simulink model "Mdl_Dim"  (R2024b)
settings: Solver=FixedStepDiscrete  StartTime=0.0  StopTime=10.0  FixedStep=0.1  RelTol=1e-3  EnableMultiTasking=on
values from neighbouring files (symbols this model uses):
  DEFAULT_MODE = mpt.Parameter    [Mdl_Dim_DD.m]
  DEFAULT_STEP = mpt.Parameter    [Mdl_Dim_DD.m]
  Mdl_Dim_cTaskPeriod = mpt.Parameter    [Mdl_Dim_rte_types.m]
  RTE_E_MAX_AGE_EXCEEDED = mpt.Parameter    [Mdl_Dim_rte_types.m]
  RTE_E_NEVER_RECEIVED = mpt.Parameter    [Mdl_Dim_rte_types.m]
  STATUS_OFF = mpt.Parameter    [Mdl_Dim_DD.m]
  STATUS_ON = mpt.Parameter    [Mdl_Dim_DD.m]
  SWITCHING_MECHANISM = mpt.Parameter    [Mdl_Dim_DD.m]
  ZERO_VAL = mpt.Parameter    [Mdl_Dim_DD.m]
undefined symbols (not defined in the file or in its folder): AppModule, CAN_COMUN_ACTIVE, CAN_COMUN_FAIL, CAN_VAL_OFF, CAN_VAL_ON, ChannelID, CLUSTER_ACTIVE, DAYNIGHT_STS_NOTRequire, DIAG_NCTRL, DIM_DAY_MODE, DIM_NIGHT_MODE, DOWN_THRESH_1SW, DrvRec_Rheo_down_Long_Press, DrvRec_Rheo_down_Short_Press, DrvRec_Rheo_up_Long_Press, DrvRec_Rheo_Up_Short_Press, DW_EVENT, DW_ON, eAppMdl_type_instance, eDayNightModeIn, eIllumination_levelIn, eSIGNAL_MISSING, eSIGNAL_NEVER_RECEIVED, eSleepSt_type_instance, FALSE, GetPwmDirect, GetPwmWithTime, GetPwmWithTimeExp, IgnOn, INDEX_MCUID0340, INDEX_MCUID0341, INDEX_MCUID0430, IoHwAb_PwmSignalIdType_type_instance, l_Wheel_Down_ParamArray, l_Wheel_Up_ParamArray, MAX_UINT16, MAXHOLD, MINHOLD, NETWORK_NORMAL, NETWORK_SLEEP, NETWORK_STANDALONE, NONE, NVM_Adapter_SetNVM_RheostatDayStep, NVM_Adapter_SetNVM_RheostatDayStepU1, NVM_Adapter_SetNVM_RheostatDayStepU2, NVM_Adapter_SetNVM_RheostatDayStepU3, NVM_Adapter_SetNVM_RheostatNightStep, NVM_Adapter_SetNVM_RheostatNightStepU1, NVM_Adapter_SetNVM_RheostatNightStepU2, NVM_Adapter_SetNVM_RheostatNightStepU3, OpeModeRheostatChange, pJustRcvdStatus, pNvmData, POS_MAX, POS_MIN, RHEO_1SW_TYPE, RHEO_2SW_TYPE, RHEO_SOFTSW_TYPE, RHEO_VALUE_FIVE_U16, RHEO_VALUE_ONE_BOOL ... (+48)
libraries: simulink x65
(part 4 of 4)

== matlab function Mdl_Dim/Mdl_Dim_Task_sys/Subsystem/Input_Process/Switch Type//2 Switch Type//Soft Switch Type/RHEO_1SW_TYPE_AND_RHEO_2SW_TYPE/Rheostat Switch Status Determination ==
  data: RHUP_Dbc_Status input; RheostatCond input; RHDW_Dbc_Status input; RheostatSwstatus output uint8; STATE_ON parameter; UP_ON parameter; Prevrheoswstatus input; VAL_ON parameter; VAL_OFF parameter; DW_ON parameter; IgnOn parameter; STATE_OFF parameter; UNKNOWN parameter; UNKNOWNSTATUS parameter; TRUE parameter; FALSE parameter
function RheostatSwstatus = fcn(RHUP_Dbc_Status, RheostatCond, RHDW_Dbc_Status, STATE_ON, UP_ON, Prevrheoswstatus, VAL_ON, VAL_OFF, DW_ON, IgnOn, STATE_OFF, UNKNOWN, UNKNOWNSTATUS, TRUE, FALSE)

aVarTruthTableCondition_1 = false;
aVarTruthTableCondition_2 = false;
aVarTruthTableCondition_3 = false;


% condition 2

aVarTruthTableCondition_1 = logical(( (RheostatCond == TRUE) && (RHUP_Dbc_Status == STATE_OFF) && (RHDW_Dbc_Status == STATE_OFF) ));

% condition 6

aVarTruthTableCondition_2 = logical(( (RheostatCond == TRUE) && (RHUP_Dbc_Status == STATE_ON) && ((Prevrheoswstatus == VAL_OFF) || (Prevrheoswstatus == UP_ON) || (Prevrheoswstatus == DW_ON)) ));

% condition 7

aVarTruthTableCondition_3 = logical(( (RheostatCond == TRUE) && (RHUP_Dbc_Status == STATE_OFF) && (RHDW_Dbc_Status == STATE_ON) && ((Prevrheoswstatus == VAL_OFF) || (Prevrheoswstatus == UP_ON) || (Prevrheoswstatus == DW_ON)) ));

if (aVarTruthTableCondition_1)
    aFcnTruthTableAction_2();
elseif (aVarTruthTableCondition_2)
    aFcnTruthTableAction_3();
elseif (aVarTruthTableCondition_3)
    aFcnTruthTableAction_4();
else % Default
    aFcnTruthTableAction_1();
end

function aFcnTruthTableAction_1()

% RhesostatSwitch status

RheostatSwstatus = UNKNOWNSTATUS;

function aFcnTruthTableAction_2()

% RhesostatSwitch status

RheostatSwstatus = VAL_OFF;

function aFcnTruthTableAction_3()

% RhesostatSwitch status

RheostatSwstatus = UP_ON;

function aFcnTruthTableAction_4()

% RhesostatSwitch status

RheostatSwstatus = DW_ON;

== matlab function Mdl_Dim/Mdl_Dim_Task_sys/Subsystem/Input_Process/Switch Type//2 Switch Type//Soft Switch Type/Night_Rheostat_Step_Determination ==
  data: Day_Night_status input; RheostatUpEvent input; RheostatDwEvent input; DIM_DAY_MODE parameter; DIM_NIGHT_MODE parameter; RTE_E_MAX_AGE_EXCEEDED parameter; MINHOLD parameter; MAXHOLD parameter; NVM_RheostatNightStep output; Prev_NVM_RheostatDayStep input; UP_EVENT parameter; NONE parameter; DW_EVENT parameter; NightChangeStatus output; TailStatus input; Get_RheostatNightStep_Val input; TRUE parameter; FALSE parameter; MCUID0341 data_store_memory
function [NVM_RheostatNightStep, NightChangeStatus] = fcn(Day_Night_status, RheostatUpEvent, RheostatDwEvent, DIM_DAY_MODE, DIM_NIGHT_MODE, RTE_E_MAX_AGE_EXCEEDED, MINHOLD, MAXHOLD, Prev_NVM_RheostatDayStep, UP_EVENT, NONE, DW_EVENT, TailStatus, Get_RheostatNightStep_Val, TRUE, FALSE)

aVarTruthTableCondition_1 = false;
aVarTruthTableCondition_2 = false;
aVarTruthTableCondition_3 = false;
aVarTruthTableCondition_4 = false;
aVarTruthTableCondition_5 = false;
aVarTruthTableCondition_6 = false;
aVarTruthTableCondition_7 = false;
aVarTruthTableCondition_8 = false;


% Night status, Up_Event and
% NVM night step >= MAXHOLD(21)

aVarTruthTableCondition_1 = logical(((Day_Night_status  == DIM_NIGHT_MODE) && (RheostatUpEvent == UP_EVENT) && (Get_RheostatNightStep_Val >= MAXHOLD)));

% Night status,Up_Event and NVM night step < MAXHOLD(21)

aVarTruthTableCondition_2 = logical(((Day_Night_status  == DIM_NIGHT_MODE) && (RheostatUpEvent == UP_EVENT) && (Get_RheostatNightStep_Val < MAXHOLD)));

% Night status,DW_Event and NVM night step = 0

aVarTruthTableCondition_3 = logical(((Day_Night_status  == DIM_NIGHT_MODE) && (RheostatUpEvent == NONE) && (RheostatDwEvent == DW_EVENT)&& (Get_RheostatNightStep_Val == MINHOLD)));

% Night status,DW_Event and NVM night step > 0

aVarTruthTableCondition_4 = logical(((Day_Night_status  == DIM_NIGHT_MODE) && (RheostatUpEvent == NONE) && (RheostatDwEvent == DW_EVENT)&& (Get_RheostatNightStep_Val > MINHOLD)));

% Day status, Up_Event and
% NVM night step >= MAXHOLD(21)

aVarTruthTableCondition_5 = logical(((Day_Night_status  == DIM_DAY_MODE) &&(MCUID0341  == TRUE) &&  (TailStatus  == TRUE) && (RheostatUpEvent == UP_EVENT) && (Get_RheostatNightStep_Val >= MAXHOLD)));

% Day status,Up_Event and NVM night step < MAXHOLD(21)

aVarTruthTableCondition_6 = logical(((Day_Night_status  == DIM_DAY_MODE)&&(MCUID0341  == TRUE) &&  (TailStatus  == TRUE) && (RheostatUpEvent == UP_EVENT) && (Get_RheostatNightStep_Val < MAXHOLD)));

% Day status,DW_Event and NVM night step = 0

aVarTruthTableCondition_7 = logical(((Day_Night_status  == DIM_DAY_MODE)  &&(MCUID0341  == TRUE) &&  (TailStatus  == TRUE) && (RheostatUpEvent == NONE) && (RheostatDwEvent == DW_EVENT)&& (Get_RheostatNightStep_Val == MINHOLD)));

% Day status,DW_Event and NVM night step > 0

aVarTruthTableCondition_8 = logical(((Day_Night_status  == DIM_DAY_MODE) &&(MCUID0341  == TRUE) &&  (TailStatus  == TRUE) && (RheostatUpEvent == NONE) && (RheostatDwEvent == DW_EVENT)&& (Get_RheostatNightStep_Val > MINHOLD)));

if (aVarTruthTableCondition_1)
    aFcnTruthTableAction_1();
elseif (aVarTruthTableCondition_2)
    aFcnTruthTableAction_2();
elseif (aVarTruthTableCondition_3)
    aFcnTruthTableAction_3();
elseif (aVarTruthTableCondition_4)
    aFcnTruthTableAction_4();
elseif (aVarTruthTableCondition_5)
    aFcnTruthTableAction_1();
elseif (aVarTruthTableCondition_6)
    aFcnTruthTableAction_2();
elseif (aVarTruthTableCondition_7)
    aFcnTruthTableAction_3();
elseif (aVarTruthTableCondition_8)
    aFcnTruthTableAction_4();
else % Default
    aFcnTruthTableAction_5();
end

function aFcnTruthTableAction_1()

    % NVM_RheostatDayStep

    NVM_RheostatNightStep = MAXHOLD;
    NightChangeStatus = FALSE;

function aFcnTruthTableAction_2()

    % NVM_RheostatDayStep

    NVM_RheostatNightStep = Prev_NVM_RheostatDayStep +1;
    NightChangeStatus = TRUE;

function aFcnTruthTableAction_3()

    % NVM_RheostatDayStep

    NVM_RheostatNightStep = MINHOLD
    NightChangeStatus = FALSE;

function aFcnTruthTableAction_4()

    % NVM_RheostatDayStep

    NVM_RheostatNightStep = Prev_NVM_RheostatDayStep-1;
    NightChangeStatus = TRUE;

function aFcnTruthTableAction_5()


    NVM_RheostatNightStep = Prev_NVM_RheostatDayStep;
    NightChangeStatus = FALSE;

== matlab function Mdl_Dim/Mdl_Dim_Task_sys/Subsystem/Input_Process/Switch Type//2 Switch Type//Soft Switch Type/RHEO_1SW_TYPE_AND_RHEO_2SW_TYPE/Subsystem/Truth Table ==
  data: RHUP_RawIn_Val output; RHEO_SW_IN_ADIN_Val input; RHDW_RawIn_Val output; VAL_ONE parameter; UP_THRESH_1SW parameter; DOWN_THRESH_1SW parameter; TRUE parameter; FALSE parameter
function [RHUP_RawIn_Val, RHDW_RawIn_Val] = fcn(RHEO_SW_IN_ADIN_Val, VAL_ONE, UP_THRESH_1SW, DOWN_THRESH_1SW, TRUE, FALSE)

aVarTruthTableCondition_1 = false;
aVarTruthTableCondition_2 = false;


% UP ON condition

aVarTruthTableCondition_1 = logical((RHEO_SW_IN_ADIN_Val < UP_THRESH_1SW));

% Down ON condition

aVarTruthTableCondition_2 = logical(( (RHEO_SW_IN_ADIN_Val >= UP_THRESH_1SW) && (RHEO_SW_IN_ADIN_Val < DOWN_THRESH_1SW)));

if (aVarTruthTableCondition_1)
    aFcnTruthTableAction_1();
elseif (aVarTruthTableCondition_2)
    aFcnTruthTableAction_2();
else % Default
    aFcnTruthTableAction_3();
end

function aFcnTruthTableAction_1()

% UP ON state

RHUP_RawIn_Val = TRUE;
RHDW_RawIn_Val = FALSE;

function aFcnTruthTableAction_2()

% DW ON state

RHDW_RawIn_Val = TRUE;
RHUP_RawIn_Val = FALSE;

function aFcnTruthTableAction_3()

% UP and DW OFF state

RHDW_RawIn_Val = FALSE;
RHUP_RawIn_Val = FALSE;

== matlab function Mdl_Dim/Mdl_Dim_Task_sys/Subsystem/Input_Process/Thumb Wheel Type/Rheostat_Step_Determination ==
  data: RheostatCond_state input; l_Wheel_RheostatStep data_store_memory; l_Wheel_RheostatChange data_store_memory; RHEO_WHEEL_STEP_INVALID parameter; RHEO_WHEEL_POS_UNDECIDED parameter; WheelPosition input; VAL_ZERO parameter; VAL_ONE parameter; l_WheelVolRatioMon_u8 data_store_memory; VAL_UNDECIDED parameter; l_AveWheelVolRaitoVal_u8 input
function fcn(RheostatCond_state, RHEO_WHEEL_STEP_INVALID, RHEO_WHEEL_POS_UNDECIDED, WheelPosition, VAL_ZERO, VAL_ONE, VAL_UNDECIDED, l_AveWheelVolRaitoVal_u8)

aVarTruthTableCondition_1 = false;
aVarTruthTableCondition_2 = false;
aVarTruthTableCondition_3 = false;


% RheostatStep is INVALID and Wheel Position Undecided

aVarTruthTableCondition_1 = logical((l_Wheel_RheostatStep == RHEO_WHEEL_STEP_INVALID) && (WheelPosition ==RHEO_WHEEL_POS_UNDECIDED));

% RheostatStep is INVALID and Wheel Position not equal to Undecided

aVarTruthTableCondition_2 = logical((l_Wheel_RheostatStep == RHEO_WHEEL_STEP_INVALID) && (WheelPosition ~=RHEO_WHEEL_POS_UNDECIDED));

% RheostatStep not equal to INVALID and Wheel Position not equal to Undecided

aVarTruthTableCondition_3 = logical((RheostatCond_state == VAL_ONE) && (l_Wheel_RheostatStep ~= RHEO_WHEEL_STEP_INVALID) && (WheelPosition ~= l_Wheel_RheostatStep));

if (aVarTruthTableCondition_1)
    aFcnTruthTableAction_1();
elseif (aVarTruthTableCondition_2)
    aFcnTruthTableAction_2();
elseif (aVarTruthTableCondition_3)
    aFcnTruthTableAction_3();
else % Default
    aFcnTruthTableAction_4();
end

function aFcnTruthTableAction_1()

% RheostatStep is INVALID and RheostatChange False

l_Wheel_RheostatStep = RHEO_WHEEL_STEP_INVALID;
l_Wheel_RheostatChange = VAL_ZERO;

function aFcnTruthTableAction_2()

% RheostatStep is Valid and RheostatChange False

l_Wheel_RheostatStep = WheelPosition;
l_Wheel_RheostatChange = VAL_ZERO;
l_WheelVolRatioMon_u8 = VAL_UNDECIDED;

function aFcnTruthTableAction_3()

% RheostatStep is Valid and RheostatChange true

l_Wheel_RheostatStep = WheelPosition;
l_Wheel_RheostatChange = VAL_ONE;
l_WheelVolRatioMon_u8 = l_AveWheelVolRaitoVal_u8;

function aFcnTruthTableAction_4()

% No Change

l_Wheel_RheostatStep = l_Wheel_RheostatStep;
l_Wheel_RheostatChange = VAL_ZERO;
l_WheelVolRatioMon_u8 = l_AveWheelVolRaitoVal_u8;

== matlab function Mdl_Dim/Mdl_Dim_Task_sys/Subsystem/Input_Process/Subsystem/Rheostat_Control_Enable_Condition_Determination ==
  data: TFTDisplayOn input; Ignstatus input; TailStatus_Val input; DIM_NIGHT_MODE parameter; RheostatCond_state output; TFT_DISPLAY_ON parameter; UNKNOWNSTATUS parameter; VAL_OFF parameter; DAYNIGHT_STS_NOTRequire parameter; IlumDayNightStatus input; DIM_DAY_MODE parameter; VAL_ON parameter; IgnOn parameter; TRUE parameter; FALSE parameter
function RheostatCond_state = fcn(TFTDisplayOn, Ignstatus, TailStatus_Val, DIM_NIGHT_MODE, TFT_DISPLAY_ON, UNKNOWNSTATUS, VAL_OFF, DAYNIGHT_STS_NOTRequire, IlumDayNightStatus, DIM_DAY_MODE, VAL_ON, IgnOn, TRUE, FALSE)

aVarTruthTableCondition_1 = false;


% Day Mode Check with CAN Missing State

aVarTruthTableCondition_1 = logical((((IlumDayNightStatus ==DIM_DAY_MODE) || (IlumDayNightStatus ==DIM_NIGHT_MODE)) && ((Ignstatus == IgnOn)|| (TFTDisplayOn ==TFT_DISPLAY_ON) || (TailStatus_Val ==VAL_ON))));

if (aVarTruthTableCondition_1)
    aFcnTruthTableAction_1();
else % Default
    aFcnTruthTableAction_2();
end

function aFcnTruthTableAction_1()

% IlumDayNightRequired is True

RheostatCond_state = TRUE;

function aFcnTruthTableAction_2()

% IlumDayNightRequired is False

RheostatCond_state = FALSE;

== matlab function Mdl_Dim/Mdl_Dim_Task_sys/Subsystem/Input_Process/Switch Type//2 Switch Type//Soft Switch Type/Day_Rheostat_Step_Determination ==
  data: Day_Night_status input; RheostatUpEvent input; RheostatDwEvent input; IgnOn parameter; DIM_DAY_MODE parameter; DIM_NIGHT_MODE parameter; RTE_E_MAX_AGE_EXCEEDED parameter; RTE_E_NEVER_RECEIVED parameter; MINHOLD parameter; MAXHOLD parameter; Get_RheostatDayStep_Val input; NVM_RheostatDayStep output; Prev_NVM_RheostatDayStep input; UP_EVENT parameter; NONE parameter; DW_EVENT parameter; DayChangeStatus output; TRUE parameter; FALSE parameter
function [NVM_RheostatDayStep, DayChangeStatus] = fcn(Day_Night_status, RheostatUpEvent, RheostatDwEvent, IgnOn, DIM_DAY_MODE, DIM_NIGHT_MODE, RTE_E_MAX_AGE_EXCEEDED, RTE_E_NEVER_RECEIVED, MINHOLD, MAXHOLD, Get_RheostatDayStep_Val, Prev_NVM_RheostatDayStep, UP_EVENT, NONE, DW_EVENT, TRUE, FALSE)

aVarTruthTableCondition_1 = false;
aVarTruthTableCondition_2 = false;
aVarTruthTableCondition_3 = false;
aVarTruthTableCondition_4 = false;


% Up_Event

aVarTruthTableCondition_1 = logical(((Day_Night_status  == DIM_DAY_MODE) && (RheostatUpEvent == UP_EVENT) && (Get_RheostatDayStep_Val >= MAXHOLD)));

% Day Mode Check with CAN Missing State

aVarTruthTableCondition_2 = logical(((Day_Night_status  == DIM_DAY_MODE) && (RheostatUpEvent == UP_EVENT) && (Get_RheostatDayStep_Val < MAXHOLD)));

% Day Mode Check with Valid Value

aVarTruthTableCondition_3 = logical(((Day_Night_status  == DIM_DAY_MODE) && (RheostatUpEvent == NONE) && (RheostatDwEvent == DW_EVENT)&& (Get_RheostatDayStep_Val == MINHOLD)));

% Day Mode Check

aVarTruthTableCondition_4 = logical(((Day_Night_status  == DIM_DAY_MODE) && (RheostatUpEvent == NONE) && (RheostatDwEvent == DW_EVENT)&& (Get_RheostatDayStep_Val > MINHOLD)));

if (aVarTruthTableCondition_1)
    aFcnTruthTableAction_1();
elseif (aVarTruthTableCondition_2)
    aFcnTruthTableAction_2();
elseif (aVarTruthTableCondition_3)
    aFcnTruthTableAction_3();
elseif (aVarTruthTableCondition_4)
    aFcnTruthTableAction_4();
else % Default
    aFcnTruthTableAction_5();
end

function aFcnTruthTableAction_1()

    % NVM_RheostatDayStep

    NVM_RheostatDayStep = MAXHOLD;
    DayChangeStatus = FALSE;

function aFcnTruthTableAction_2()

    % NVM_RheostatDayStep

    NVM_RheostatDayStep = Prev_NVM_RheostatDayStep +1;
    DayChangeStatus = TRUE;

function aFcnTruthTableAction_3()

    % NVM_RheostatDayStep

    NVM_RheostatDayStep = MINHOLD;
    DayChangeStatus = FALSE;

function aFcnTruthTableAction_4()

    % NVM_RheostatDayStep

    NVM_RheostatDayStep = Prev_NVM_RheostatDayStep-1;
    DayChangeStatus = TRUE;

function aFcnTruthTableAction_5()


    NVM_RheostatDayStep = Prev_NVM_RheostatDayStep;
    DayChangeStatus = FALSE;
